simulink model "software2"  (Simulink 7.4)
settings: Solver=ode45  StartTime=0.0  StopTime=2  RelTol=1e-3
libraries: dspxfrm3 x1, dspsrcs4 x1
settings Model: Creator=Chris  LastModifiedBy=Chris
settings SimEventsCC: propDiagAttribOutput=1  propDiagFcnCallOutput=1  propDiagStatOutput=0

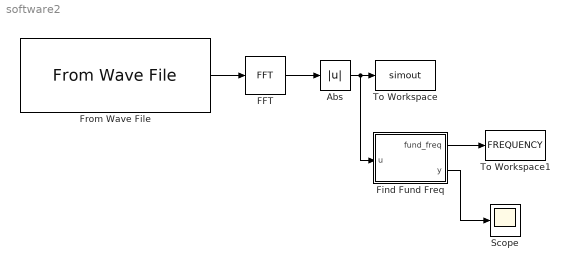
== system software2 ==
  Abs : Abs  OutDataTypeMode=double  OutDataType=fixdt(1, 16)  OutScaling=2^0  OutDataTypeStr=double
  FFT : dspxfrm3/FFT  DialogController=dspDDGCreate  DialogControllerArgs=DataTag0  CompMethod=Table lookup  TableOpt=NEW  TableOptActive=Speed  BitRevOrder=off  InheritFFTLength=on  FFTLength=64  SkipNorm=off  roundingMode=Floor  overflowMode=off
  Find Fund Freq : Stateflow chart
  From Wave File : dspsrcs4/From Wave File  FileName=test5_789_8192sample.wav  SamplesPerFrame=8192  MinBufSize=8192  dType=double  bLoop=off  timesToPlay=1  restartMode=immediately after last sample  firstSampleOutput=off  lastSampleOutput=off
  Scope : Scope
  To Workspace : ToWorkspace  VariableName=simout  SampleTime=-1  SaveFormat=Array
  To Workspace1 : ToWorkspace  VariableName=FREQUENCY  SampleTime=-1  SaveFormat=Array
  wires:
  FFT/1 -> Abs/1
  Abs/1 -> To Workspace/1, Find Fund Freq/1(u)
  From Wave File/1 -> FFT/1
  Find Fund Freq/2(y) -> Scope/1
  Find Fund Freq/1(fund_freq) -> To Workspace1/1

== matlab function Find Fund Freq ==
  data: u input double; fund_freq output double size=1,1 [0..99999999]; y output double
function [fund_freq, y]= fcn(u)
%#em2
%Chris Jagielski
%Find Fundamental Frequency!

y = u; %retain spectrum

value = max(u); %peak in frequency domain
a = find(u==value,1,'first')-1; %finds only 1 value that matches
fund_freq = a(1,1);
